simulink model "linearizzato"  (R2020b)
settings: Solver=FixedStepAuto  StartTime=0.0  StopTime=100.0  FixedStep=0.02  RelTol=1e-3
values from neighbouring files (symbols this model uses):
  U = sqrt(x(1)^2 + x(2)^2)    [shipLIN_Sfun.m]    (also in shipNL_Sfun.m)
  X = Xh + Xr + Xp    [shipLIN_Sfun.m]    (also in shipNL_Sfun.m)
  Y = Yh + Yr    [shipLIN_Sfun.m]    (also in shipNL_Sfun.m)
undefined symbols (not defined in the file or in its folder): A, B, C, D, p
settings Model: Creator=teora  LastModifiedBy=teora

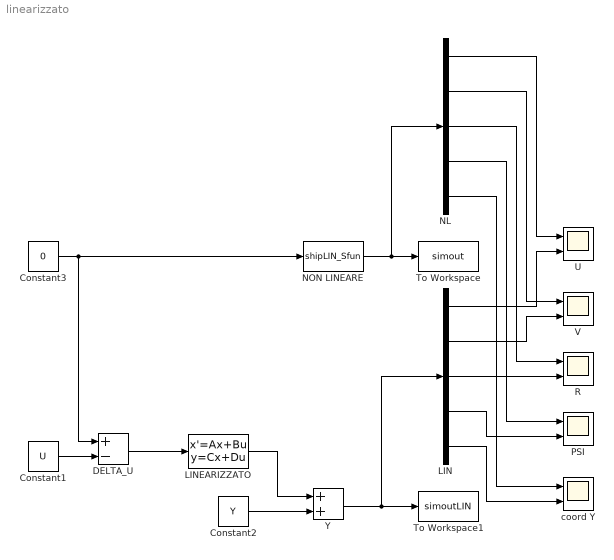
== system linearizzato ==
  Constant1 : Constant  Value=U
  Constant2 : Constant  Value=Y
  Constant3 : Constant  Value=0
  DELTA_U : Sum  Inputs=+-
  LIN : Demux  Outputs=5
  LINEARIZZATO : StateSpace  A=A  B=B  C=C  D=D  InitialCondition=[0;0;0;0;0]
  NL : Demux  Outputs=5
  NON LINEARE : S-Function  FunctionName=shipLIN_Sfun  Parameters=p,X  SFunctionDeploymentMode=off  EnableBusSupport=off
  PSI : Scope  NumInputPorts=2
  R : Scope  NumInputPorts=2
  To Workspace : ToWorkspace  VariableName=simout  SaveFormat=Timeseries  SampleTime=-1
  To Workspace1 : ToWorkspace  VariableName=simoutLIN  SaveFormat=Timeseries  SampleTime=-1
  U : Scope  NumInputPorts=2
  V : Scope  NumInputPorts=2
  Y : Sum
  coord Y : Scope  NumInputPorts=2
  wires:
  DELTA_U/1 -> LINEARIZZATO/1
  Constant1/1 -> DELTA_U/2
  NON LINEARE/1 -> To Workspace/1, NL/1
  LINEARIZZATO/1 -> Y/1
  Constant2/1 -> Y/2
  NL/3 -> R/1
  NL/1 -> U/1
  NL/2 -> V/1
  LIN/2 -> V/2
  NL/4 -> PSI/1
  LIN/4 -> PSI/2
  Constant3/1 -> DELTA_U/1, NON LINEARE/1
  LIN/1 -> U/2
  LIN/5 -> coord Y/2
  LIN/3 -> R/2
  NL/5 -> coord Y/1
  Y/1 -> To Workspace1/1, LIN/1
